simulink model "twolink_inv"  (R2017b)
settings: Solver=VariableStepAuto  StartTime=0.0  StopTime=20  RelTol=1e-3
values from neighbouring files (symbols this model uses):
  h = diff(x)    [dfdx.m]    (also in inv_control.m = -m2*l1*lc2*sin(q2); twolink_ftraj.m = 0.1; twolink_valid.m = 0.1)
libraries: roblocks x1
settings Model: Creator=sathish  LastModifiedBy=sathish

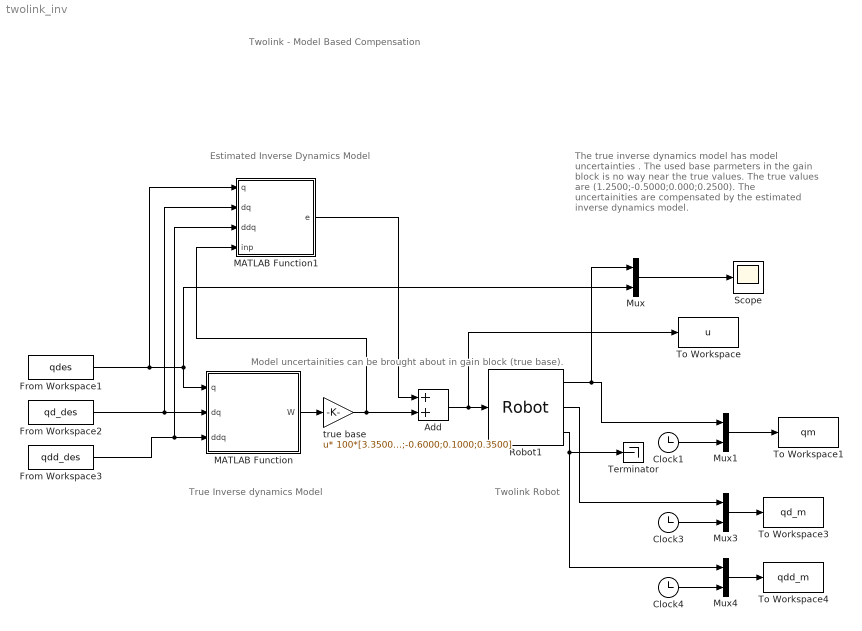
== system twolink_inv ==
  note: The true inverse dynamics model has model uncertainties . The used base parmeters in the gain block is no way near the true values. The true values are (1.2500;-0.5000;0.000;0.2500). The uncertainities are compensated by the estimated inverse dynamics model.
  note: Model uncertainities can be brought about in gain block (true base).
  note: Twolink Robot
  note: True Inverse dynamics Model
  note: Estimated Inverse Dynamics Model
  note: Twolink - Model Based Compensation
  Add : Sum
  Clock1 : Clock
  Clock3 : Clock
  Clock4 : Clock
  From Workspace1 : FromWorkspace  VariableName=qdes  SampleTime=0
  From Workspace2 : FromWorkspace  VariableName=qd_des  SampleTime=0
  From Workspace3 : FromWorkspace  VariableName=qdd_des  SampleTime=0
  MATLAB Function : MATLAB Function  TreatAsAtomicUnit=on
  MATLAB Function1 : MATLAB Function  TreatAsAtomicUnit=on
  Mux{,1,3..4} (4 alike) : Mux  Inputs=2
  Robot1 : roblocks/Arm/Robot  robot=twolink_mod  q0=[0 0]
  Scope : Scope
  Terminator : Terminator
  To Workspace : ToWorkspace  VariableName=u  SampleTime=h
      settings: Save2DSignal=2-D array (concatenate along first dimension)
  To Workspace1 : ToWorkspace  VariableName=qm  SaveFormat=Timeseries  SampleTime=h
  To Workspace3 : ToWorkspace  VariableName=qd_m  SaveFormat=Timeseries  SampleTime=h
  To Workspace4 : ToWorkspace  VariableName=qdd_m  SaveFormat=Timeseries  SampleTime=h
  true base : Gain  Gain=100*[3.3500;-0.6000;0.1000;0.3500]  Multiplication=Matrix(u*K)
  wires:
  Mux1/1 -> To Workspace1/1
  Robot1/2 -> Mux3/1
  Robot1/1 -> Mux1/1, Mux/1
  Clock1/1 -> Mux1/2
  Mux4/1 -> To Workspace4/1
  Clock3/1 -> Mux3/2
  Robot1/3 -> Mux4/1, Terminator/1
  Mux/1 -> Scope/1
  Clock4/1 -> Mux4/2
  Mux3/1 -> To Workspace3/1
  MATLAB Function/1(W) -> true base/1
  From Workspace2/1 -> MATLAB Function1/2(dq), MATLAB Function/2(dq)
  From Workspace3/1 -> MATLAB Function1/3(ddq), MATLAB Function/3(ddq)
  From Workspace1/1 -> MATLAB Function1/1(q), MATLAB Function/1(q), Mux/2
  true base/1 -> MATLAB Function1/4(inp), Add/2
  MATLAB Function1/1(e) -> Add/1
  Add/1 -> To Workspace/1, Robot1/1

== matlab function twolink_inv/MATLAB Function1 ==
  data: q input; e output; dq input; ddq input; inp input
function e = Regressor(q,dq,ddq,inp)
x0 = ((dq(1))*(dq(1)));
x1 = ddq(1) + ddq(2);
x2 = sin(q(2));
x3 = dq(1)*x2;
x4 = dq(1) + dq(2);
x5 = cos(q(2));
x6 = ddq(1)*x5 - dq(2)*x3 + x3*x4;
x7 = -((x4)*(x4));
x8 = dq(1)*x5;
x9 = ddq(1)*x2 + dq(2)*x8;
x10 = x4*x8;
x11 = x10 - x9;
H = zeros(2,20);
  H(1) = 0;
  H(2) = 0;
  H(3) = 0;
  H(4) = 0;
  H(5) = 0;
  H(6) = ddq(1);
  H(7) = 2*ddq(1);
  H(8) = 0;
  H(8) = 0;
  H(10) = ddq(1);
  H(11) = 0;
  H(12) = 0;
  H(13) = 0;
  H(14) = 0;
  H(15) = 0;
  H(16) = x1;
  H(17) = x1*x5 + x2*x7 + x6;
  H(18) = -x1*x2 + x11 + x5*x7;
  H(19) = 0;
  H(20) = x2*(-x10 + x9) + x5*x6;
  H(21) = 0;
  H(22) = 0;
  H(23) = 0;
  H(24) = 0;
  H(25) = 0;
  H(26) = 0;
  H(27) = 0;
  H(28) = 0;
  H(29) = 0;
  H(30) = 0;
  H(31) = 0;
  H(32) = 0;
  H(33) = 0;
  H(34) = 0;
  H(35) = 0;
  H(36) = x1;
  H(37) = x6;
  H(38) = x11;
  H(39) = 0;
  H(40) = 0;
  Wl = zeros(2,20);
  k = 1;
     for i = 1:2
         for j = 1:20
             Wl(i,j) = H(k); 
             k = k+1;
         end
     end
     Wb1 = Wl(:,6);
     Wb2 = Wl(:,17);
     Wb3 = Wl(:,18);
     Wb4 = Wl(:,16);
     W = [Wb1,Wb2,Wb3,Wb4];
     est = [1.2500;-0.5000;0.000;0.2500];
     V = W*est; 
     e = zeros(2,1);
     if(isequal(inp,V))
         e = [0;0];
     else
         e = V - inp;
     end
end

== matlab function twolink_inv/MATLAB Function ==
  data: q input; W output; dq input; ddq input
function W = Regressor(q,dq,ddq)
x0 = ((dq(1))*(dq(1)));
x1 = ddq(1) + ddq(2);
x2 = sin(q(2));
x3 = dq(1)*x2;
x4 = dq(1) + dq(2);
x5 = cos(q(2));
x6 = ddq(1)*x5 - dq(2)*x3 + x3*x4;
x7 = -((x4)*(x4));
x8 = dq(1)*x5;
x9 = ddq(1)*x2 + dq(2)*x8;
x10 = x4*x8;
x11 = x10 - x9;
H = zeros(2,20);
  H(1) = 0;
  H(2) = 0;
  H(3) = 0;
  H(4) = 0;
  H(5) = 0;
  H(6) = ddq(1);
  H(7) = 2*ddq(1);
  H(8) = 0;
  H(8) = 0;
  H(10) = ddq(1);
  H(11) = 0;
  H(12) = 0;
  H(13) = 0;
  H(14) = 0;
  H(15) = 0;
  H(16) = x1;
  H(17) = x1*x5 + x2*x7 + x6;
  H(18) = -x1*x2 + x11 + x5*x7;
  H(19) = 0;
  H(20) = x2*(-x10 + x9) + x5*x6;
  H(21) = 0;
  H(22) = 0;
  H(23) = 0;
  H(24) = 0;
  H(25) = 0;
  H(26) = 0;
  H(27) = 0;
  H(28) = 0;
  H(29) = 0;
  H(30) = 0;
  H(31) = 0;
  H(32) = 0;
  H(33) = 0;
  H(34) = 0;
  H(35) = 0;
  H(36) = x1;
  H(37) = x6;
  H(38) = x11;
  H(39) = 0;
  H(40) = 0;
  Wl = zeros(2,20);
  k = 1;
     for i = 1:2
         for j = 1:20
             Wl(i,j) = H(k); 
             k = k+1;
         end
     end
     Wb1 = Wl(:,6);
     Wb2 = Wl(:,17);
     Wb3 = Wl(:,18);
     Wb4 = Wl(:,16);
     W = [Wb1,Wb2,Wb3,Wb4];
end
